simulink model "Control_model_10DOF_fin"  (R2016b)
settings: Solver=FixedStepAuto  StartTime=0.0  StopTime=10  FixedStep=0.0001  RelTol=1e-3
InitFcn:
  | Initialisation_ctr_10DOF_fin
values from neighbouring files (symbols this model uses):
  COM_Parameters = [-lpelvis/2;r2;0]    [Initialisation_ctr_10DOF_fin.m]
  DH_Parameters = [hfoot 0 ... (first row only)    [Initialisation_ctr_10DOF_fin.m]
  dTrunk = trunklbd(3)    [Initialisation_ctr_10DOF_fin.m]
  dxFootSM = dxFoot    [Initialisation_ctr_10DOF_fin.m]
  dxTrunk = 0.1    [Initialisation_ctr_10DOF_fin.m]
  Foot_Parameters = [0;-(lFoot/2-lHeel);0]    [Initialisation_ctr_10DOF_fin.m]
  HAA2HEE = [0; 0; 0.001]    [Initialisation_ctr_10DOF_fin.m]
  HEE2HFE = 0.5*[0.2; 0; 0]    [Initialisation_ctr_10DOF_fin.m]
  height_vrp = CoM_position(1)    [Initialisation_ctr_10DOF_fin.m]
  hTrunk = trunklbd(1)    [Initialisation_ctr_10DOF_fin.m]
  initial_CoM_position = R*CoM_position    [Initialisation_ctr_10DOF_fin.m]
  initial_CoM_velocity = [0;0;0]    [Initialisation_ctr_10DOF_fin.m]
  initial_left_foot = [0;0;-stance_width/2]    [Initialisation_ctr_10DOF_fin.m]
  initial_right_foot = [0;0;stance_width/2]    [Initialisation_ctr_10DOF_fin.m]
  initial_RorL = 0    [Initialisation_ctr_10DOF_fin.m]
  jointsinitial = [9;-15;6;0;0;6;-15;9]/180*pi    [Initialisation_ctr_10DOF_fin.m]
  K_DCM = 4.3*[1 0 0 ... (first row only)    [Initialisation_ctr_10DOF_fin.m]
  kD_left = mbody*[0.95 0 0 0 ... (first row only)    [Initialisation_ctr_10DOF_fin.m]
  kD_right = mbody*[0.12 0 0 0 ... (first row only)    [Initialisation_ctr_10DOF_fin.m]
  kI_left = mbody*[35 0 0 0 ... (first row only)    [Initialisation_ctr_10DOF_fin.m]
  kI_right = mbody*[38.2 0 0 0 ... (first row only)    [Initialisation_ctr_10DOF_fin.m]
  kP_left = mbody*[75 0 0 0 ... (first row only)    [Initialisation_ctr_10DOF_fin.m]
  kP_right = mbody*[5.6 0 0 0 ... (first row only)    [Initialisation_ctr_10DOF_fin.m]
  Lenght = [lShank;lThigh]    [Initialisation_ctr_10DOF_fin.m]
  lFootSM = lFoot    [Initialisation_ctr_10DOF_fin.m]
  lpelvis = wPelvis    [Initialisation_ctr_10DOF_fin.m]
  mass = mbody    (= 60)    [Initialisation_ctr_10DOF_fin.m]
  Masses = [mThigh; mShank; mTrunk]    [Initialisation_ctr_10DOF_fin.m]
  nb_step = 4    [Initialisation_ctr_10DOF_fin.m]
  nb_step_pattern = 20    [Initialisation_ctr_10DOF_fin.m]
  Pelvis_Parameters = [-lpelvis/2;hTrunk/2;0]    [Initialisation_ctr_10DOF_fin.m]
  stance_width = lpelvis    [Initialisation_ctr_10DOF_fin.m]
  stride_lenght = 0.50    (= 0.5)    [Initialisation_ctr_10DOF_fin.m]
  T_DS = time_DS    (= 0.4)    [Initialisation_ctr_10DOF_fin.m]
  T_IT = time_DS    (= 0.4)    [Initialisation_ctr_10DOF_fin.m]
  T_SS = time_swing    (= 1.6)    [Initialisation_ctr_10DOF_fin.m]
  time_DS = (time_stance-time_swing)/2    (= 0.4)    [Initialisation_ctr_10DOF_fin.m]
  time_stance = 60/100*time_stride    (= 2.4)    [Initialisation_ctr_10DOF_fin.m]
  time_step = time_stride/2    (= 2)    [Initialisation_ctr_10DOF_fin.m]
  time_swing = 40/100*time_stride    (= 1.6)    [Initialisation_ctr_10DOF_fin.m]
  validity_angle = [-20*pi/180 20*pi/180 ... (first row only)    [Initialisation_ctr_10DOF_fin.m]
  wTrunk = trunklbd(2)    [Initialisation_ctr_10DOF_fin.m]
  x4CoM = CoM_position(1)-XR4(1)    [Initialisation_ctr_10DOF_fin.m]
undefined symbols (not defined in the file or in its folder): dsegment, hFoot, l, lFoot, omega0_x, omega0_z, rho, wPelvis, X, Xp_x, Xp_z, Y, Z
undefined symbols (not defined in the file): k_grf, lShankSM, lThighSM, mShank, mThigh
libraries: nesl_utility x247, sm_lib x215, dspindex x12, FootPlacementLibrary x8, dspsigops x4, dspswit3 x1
(part 1 of 18)
settings Model: Creator=Damien  LastModifiedBy=Damien

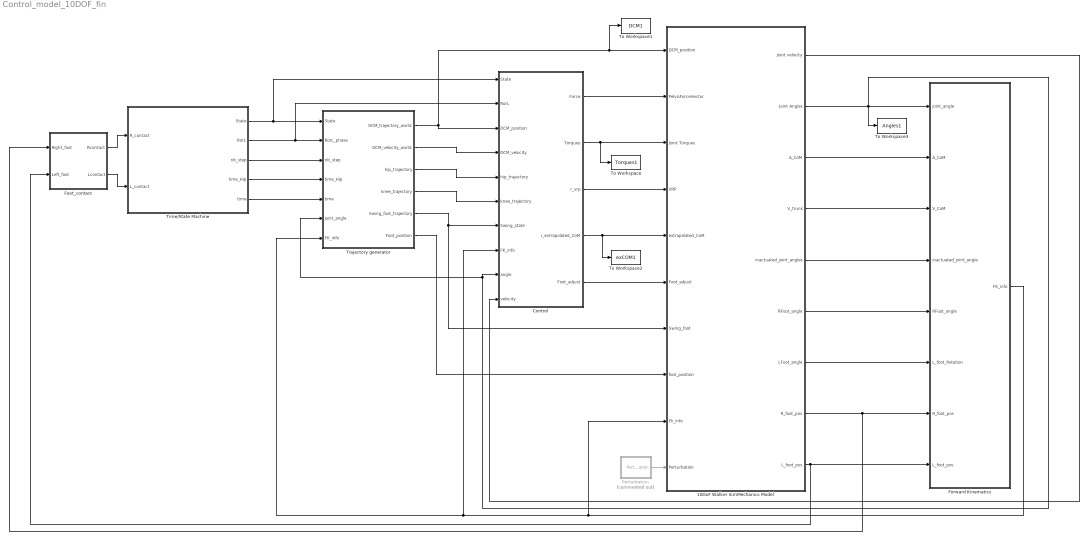
== system Control_model_10DOF_fin ==
  10DoF Walker SimMechanics Model : Subsystem
  Control : Subsystem
  Foot_contact : Subsystem
  Forward Kinematics : Subsystem
  Perturbation : Subsystem  Commented=on
  Time/State Machine : Subsystem
  To Workspace : ToWorkspace  VariableName=Torques1  SaveFormat=Timeseries  SampleTime=-1
  To Workspace1 : ToWorkspace  VariableName=DCM1  SaveFormat=Timeseries  SampleTime=-1
  To Workspace2 : ToWorkspace  VariableName=exCOM1  SaveFormat=Timeseries  SampleTime=-1
  To Workspace3 : ToWorkspace  VariableName=Angles1  SaveFormat=Timeseries  SampleTime=-1
  Trajectory generator : Subsystem
  wires:
  10DoF Walker SimMechanics Model/1(Joint velocity) -> Control/10(velocity)
  10DoF Walker SimMechanics Model/2(Joint Angles) -> Trajectory generator/6(joint_angle), Control/9(angle), To Workspace3/1, Forward Kinematics/1(joint_angle)
  Forward Kinematics/1(FK_info) -> Trajectory generator/7(FK_info), Control/8(FK_info), 10DoF Walker SimMechanics Model/9(Fk_info)
  10DoF Walker SimMechanics Model/4(V_trunk) -> Forward Kinematics/3(V_CoM)
  10DoF Walker SimMechanics Model/6(RFoot_angle) -> Forward Kinematics/5(RFoot_angle)
  10DoF Walker SimMechanics Model/3(A_CoM) -> Forward Kinematics/2(A_CoM)
  10DoF Walker SimMechanics Model/8(R_foot_pos) -> Foot_contact/1(Right_foot), Forward Kinematics/7(R_foot_pos)
  Trajectory generator/5(Swing_foot_trajectory) -> 10DoF Walker SimMechanics Model/7(Swing_foot), Control/7(Swing_state)
  Trajectory generator/1(DCM_trajectory_world) -> To Workspace1/1, 10DoF Walker SimMechanics Model/1(DCM_position), Control/3(DCM_position)
  Trajectory generator/6(Foot_position) -> 10DoF Walker SimMechanics Model/8(foot_position)
  Trajectory generator/2(DCM_velocity_world) -> Control/4(DCM_velocity)
  10DoF Walker SimMechanics Model/7(LFoot_angle) -> Forward Kinematics/6(L_foot_Rotation)
  10DoF Walker SimMechanics Model/9(L_foot_pos) -> Foot_contact/2(Left_foot), Forward Kinematics/8(L_foot_pos)
  10DoF Walker SimMechanics Model/5(inactuated_joint_angles) -> Forward Kinematics/4(inactuated_joint_angle)
  Control/2(Torques) -> 10DoF Walker SimMechanics Model/3(Joint Torques), To Workspace/1
  Control/1(Force) -> 10DoF Walker SimMechanics Model/2(PelvisForceVector)
  Control/3(r_vrp) -> 10DoF Walker SimMechanics Model/4(VRP)
  Control/4(r_extrapolated_CoM) -> 10DoF Walker SimMechanics Model/5(extrapolated_CoM), To Workspace2/1
  Trajectory generator/3(hip_trajectory) -> Control/5(hip_trajectory)
  Time/State Machine/2(RorL) -> Control/2(RorL), Trajectory generator/2(RorL_phase)
  Time/State Machine/3(nb_step) -> Trajectory generator/3(nb_step)
  Time/State Machine/1(State) -> Control/1(State), Trajectory generator/1(State)
  Time/State Machine/4(time_Hip) -> Trajectory generator/4(time_Hip)
  Foot_contact/1(Rcontact) -> Time/State Machine/1(R_contact)
  Foot_contact/2(Lcontact) -> Time/State Machine/2(L_contact)
  Control/5(Foot_adjust) -> 10DoF Walker SimMechanics Model/6(Foot_adjust)
  Time/State Machine/5(time) -> Trajectory generator/5(time)
  Trajectory generator/4(knee_trajectory) -> Control/6(knee_trajectory)
  Perturbation/1(Perturbation) -> 10DoF Walker SimMechanics Model/10(Perturbation)

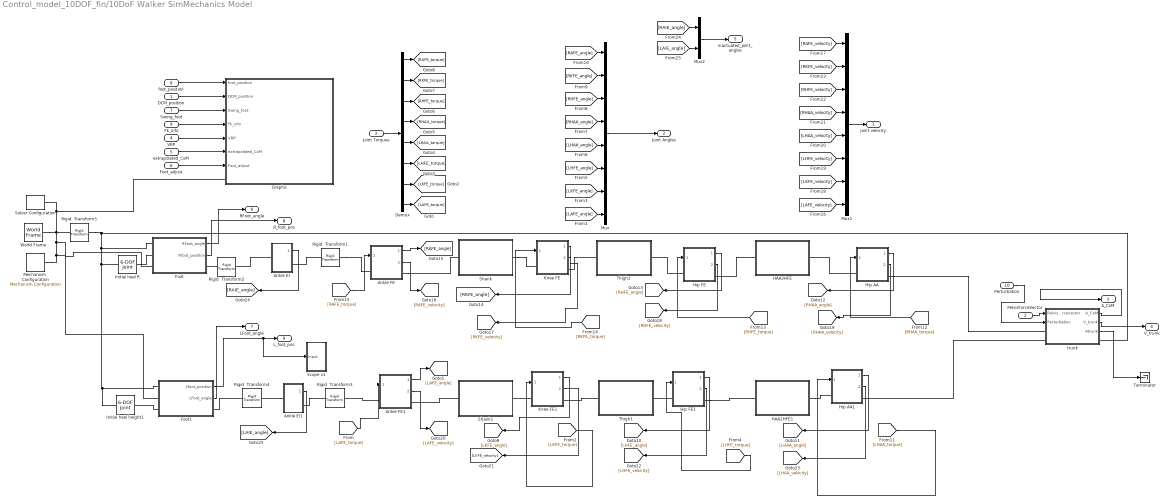
== system Control_model_10DOF_fin/10DoF Walker SimMechanics Model ==
  DCM_position : Inport
  PelvisForceVector : Inport  Port=2
  Joint Torques : Inport  Port=3  PortDimensions=8
  VRP : Inport  Port=4
  extrapolated_CoM : Inport  Port=5
  Foot_adjust : Inport  Port=6
  Swing_foot : Inport  Port=7
  foot_position : Inport  Port=8
  Fk_info : Inport  Port=9
  Perturbation : Inport  Port=10
  Ankle EI : Subsystem
  Ankle EI1 : Subsystem
  Ankle FE : Subsystem
  Ankle FE1 : Subsystem
  Demux : Demux  Outputs=8
  Foot : Subsystem  mask{l=lFootSM, k=k_grf}
      mask prompts: l "Foot length"; k "Ground contact parameters"
  Foot1 : Subsystem  mask{l=lFootSM, k=k_grf}
      mask prompts: l "Foot length"; k "Ground contact parameters"
  Graphic : Subsystem
  HAA2HFE : Subsystem
  HAA2HFE1 : Subsystem
  Hip AA : Subsystem
  Hip AA1 : Subsystem
  Hip FE : Subsystem
  Hip FE1 : Subsystem
  Initial heel R : sm_lib/Joints/6-DOF Joint  SenseConstraintForce=off  SenseConstraintForceX=off  SenseConstraintForceY=off  SenseConstraintForceZ=off  SenseConstraintTorque=off  SenseConstraintTorqueX=off  SenseConstraintTorqueY=off  SenseConstraintTorqueZ=off  SenseTotalForce=off  SenseTotalForceX=off  SenseTotalForceY=off  SenseTotalForceZ=off  SenseTotalTorque=off  SenseTotalTorqueX=off  SenseTotalTorqueY=off  SenseTotalTorqueZ=off  CompositeWrenchDir=FollowerOnBase  CompositeWrenchFrame=BaseFrame  PxEquilibriumPosition=0  PxEquilibriumPositionUnits=m  PxSpringStiffness=0  PxSpringStiffnessUnits=N/m  PxDampingCoefficient=0  PxDampingCoefficientUnits=N/(m/s)  PxTorqueActuationMode=NoTorque  PxMotionActuationMode=ComputedMotion  PxSensePosition=off  PxSenseVelocity=off  PxSenseAcceleration=off  PxSenseTorqueForce=off  PxPositionTargetSpecify=off  PxPositionTargetPriority=High  PxPositionTargetValue=0  PxPositionTargetValueUnits=m  PxVelocityTargetSpecify=off  PxVelocityTargetPriority=High  PxVelocityTargetValue=0  PxVelocityTargetValueUnits=m/s  PyEquilibriumPosition=0  PyEquilibriumPositionUnits=m  PySpringStiffness=0  PySpringStiffnessUnits=N/m  PyDampingCoefficient=0  PyDampingCoefficientUnits=N/(m/s)  PyTorqueActuationMode=NoTorque  PyMotionActuationMode=ComputedMotion  PySensePosition=off  PySenseVelocity=off  PySenseAcceleration=off  PySenseTorqueForce=off  PyPositionTargetSpecify=off  PyPositionTargetPriority=High  PyPositionTargetValue=0  PyPositionTargetValueUnits=m  PyVelocityTargetSpecify=off  PyVelocityTargetPriority=High  PyVelocityTargetValue=0  PyVelocityTargetValueUnits=m/s  PzEquilibriumPosition=0  PzEquilibriumPositionUnits=m  PzSpringStiffness=0  PzSpringStiffnessUnits=N/m  PzDampingCoefficient=0  PzDampingCoefficientUnits=N/(m/s)  PzTorqueActuationMode=NoTorque  PzMotionActuationMode=ComputedMotion  PzSensePosition=off  PzSenseVelocity=off  PzSenseAcceleration=off  PzSenseTorqueForce=off  PzPositionTargetSpecify=off  PzPositionTargetPriority=High  PzPositionTargetValue=0  PzPositionTargetValueUnits=m  PzVelocityTargetSpecify=off  PzVelocityTargetPriority=High  PzVelocityTargetValue=0  PzVelocityTargetValueUnits=m/s  SphDefPosRotationMethod=None  SphDefPosRotationAngleUnits=deg  SphDefPosRotationStandardAxis=+Z  SphDefPosRotationAngle=0  SphDefPosRotationArbitraryAxis=[0 0 1]  SphDefPosFollAlignAxisA=+X  SphDefPosBaseAlignAxisA=+Y  SphDefPosFollAlignAxisB=+Y  SphDefPosBaseAlignAxisB=+Z  SphDefPosRotationSequenceAxes=FollowerAxes  SphDefPosRotationSequence=XYX  SphDefPosRotationSequenceAngles=[0 0 0]  SphDefPosRotationSequenceAnglesUnits=deg  SphDefPosRotationMatrix=[1 0 0; 0 1 0; 0 0 1]  SphEqPosRotationMethod=None  SphEqPosRotationAngleUnits=deg  SphEqPosRotationStandardAxis=+Z  SphEqPosRotationAngle=0  SphEqPosRotationArbitraryAxis=[0 0 1]  SphEqPosFollAlignAxisA=+X  SphEqPosBaseAlignAxisA=+Y  SphEqPosFollAlignAxisB=+Y  SphEqPosBaseAlignAxisB=+Z  SphEqPosRotationSequenceAxes=FollowerAxes  SphEqPosRotationSequence=XYX  SphEqPosRotationSequenceAngles=[0 0 0]  SphEqPosRotationSequenceAnglesUnits=deg  SphEqPosRotationMatrix=[1 0 0; 0 1 0; 0 0 1]  SphSpringStiffness=0  SphSpringStiffnessUnits=N*m/deg  SphDampingCoefficient=0  SphDampingCoefficientUnits=N*m/(deg/s)  SphActuateTorqueX=off  SphActuateTorqueY=off  SphActuateTorqueZ=off  SphActuateTorque=off  SphTorqueActuationMode=NoTorque  SphMotionActuationMode=ComputedMotion  SphActuationFrame=BaseFrame  SphSensePosition=off  SphSenseVelocityX=off  SphSenseVelocityY=off  SphSenseVelocityZ=off  SphSenseVelocity=off  SphSenseAccelerationX=off  SphSenseAccelerationY=off  SphSenseAccelerationZ=off  SphSenseAcceleration=off  SphSenseTorqueX=off  SphSenseTorqueY=off  SphSenseTorqueZ=off  SphSenseTorqueForce=off  SphSensingFrame=BaseFrame  SphPositionTargetRotationMethod=None  SphPositionTargetRotationAngleUnits=deg  SphPositionTargetRotationStandardAxis=+Z  SphPositionTargetRotationAngle=0  SphPositionTargetRotationArbitraryAxis=[0 0 1]  SphPositionTargetFollAlignAxisA=+X  SphPositionTargetBaseAlignAxisA=+Y  SphPositionTargetFollAlignAxisB=+Y  SphPositionTargetBaseAlignAxisB=+Z  SphPositionTargetRotationSequenceAxes=FollowerAxes  SphPositionTargetRotationSequence=XYX  SphPositionTargetRotationSequenceAngles=[0 0 0]  SphPositionTargetRotationSequenceAnglesUnits=deg  SphPositionTargetRotationMatrix=[1 0 0; 0 1 0; 0 0 1]  SphPositionTargetSpecify=off  SphPositionTargetPriority=High  SphVelocityTargetValue=[0 0 0]  SphVelocityTargetValueUnits=deg/s  SphVelocityTargetSpecify=off  SphVelocityTargetPriority=High  SphVelocityTargetInFollowerFrame=on
  Initial heel height1 : sm_lib/Joints/6-DOF Joint  SenseConstraintForce=off  SenseConstraintForceX=off  SenseConstraintForceY=off  SenseConstraintForceZ=off  SenseConstraintTorque=off  SenseConstraintTorqueX=off  SenseConstraintTorqueY=off  SenseConstraintTorqueZ=off  SenseTotalForce=off  SenseTotalForceX=off  SenseTotalForceY=off  SenseTotalForceZ=off  SenseTotalTorque=off  SenseTotalTorqueX=off  SenseTotalTorqueY=off  SenseTotalTorqueZ=off  CompositeWrenchDir=FollowerOnBase  CompositeWrenchFrame=BaseFrame  PxEquilibriumPosition=0  PxEquilibriumPositionUnits=m  PxSpringStiffness=0  PxSpringStiffnessUnits=N/m  PxDampingCoefficient=0  PxDampingCoefficientUnits=N/(m/s)  PxTorqueActuationMode=NoTorque  PxMotionActuationMode=ComputedMotion  PxSensePosition=off  PxSenseVelocity=off  PxSenseAcceleration=off  PxSenseTorqueForce=off  PxPositionTargetSpecify=off  PxPositionTargetPriority=High  PxPositionTargetValue=0  PxPositionTargetValueUnits=m  PxVelocityTargetSpecify=off  PxVelocityTargetPriority=High  PxVelocityTargetValue=0  PxVelocityTargetValueUnits=m/s  PyEquilibriumPosition=0  PyEquilibriumPositionUnits=m  PySpringStiffness=0  PySpringStiffnessUnits=N/m  PyDampingCoefficient=0  PyDampingCoefficientUnits=N/(m/s)  PyTorqueActuationMode=NoTorque  PyMotionActuationMode=ComputedMotion  PySensePosition=off  PySenseVelocity=off  PySenseAcceleration=off  PySenseTorqueForce=off  PyPositionTargetSpecify=on  PyPositionTargetPriority=High  PyPositionTargetValue=0  PyPositionTargetValueUnits=m  PyVelocityTargetSpecify=off  PyVelocityTargetPriority=High  PyVelocityTargetValue=0  PyVelocityTargetValueUnits=m/s  PzEquilibriumPosition=0  PzEquilibriumPositionUnits=m  PzSpringStiffness=0  PzSpringStiffnessUnits=N/m  PzDampingCoefficient=0  PzDampingCoefficientUnits=N/(m/s)  PzTorqueActuationMode=NoTorque  PzMotionActuationMode=ComputedMotion  PzSensePosition=off  PzSenseVelocity=off  PzSenseAcceleration=off  PzSenseTorqueForce=off  PzPositionTargetSpecify=off  PzPositionTargetPriority=High  PzPositionTargetValue=0  PzPositionTargetValueUnits=m  PzVelocityTargetSpecify=off  PzVelocityTargetPriority=High  PzVelocityTargetValue=0  PzVelocityTargetValueUnits=m/s  SphDefPosRotationMethod=None  SphDefPosRotationAngleUnits=deg  SphDefPosRotationStandardAxis=+Z  SphDefPosRotationAngle=0  SphDefPosRotationArbitraryAxis=[0 0 1]  SphDefPosFollAlignAxisA=+X  SphDefPosBaseAlignAxisA=+Y  SphDefPosFollAlignAxisB=+Y  SphDefPosBaseAlignAxisB=+Z  SphDefPosRotationSequenceAxes=FollowerAxes  SphDefPosRotationSequence=XYX  SphDefPosRotationSequenceAngles=[0 0 0]  SphDefPosRotationSequenceAnglesUnits=deg  SphDefPosRotationMatrix=[1 0 0; 0 1 0; 0 0 1]  SphEqPosRotationMethod=None  SphEqPosRotationAngleUnits=deg  SphEqPosRotationStandardAxis=+Z  SphEqPosRotationAngle=0  SphEqPosRotationArbitraryAxis=[0 0 1]  SphEqPosFollAlignAxisA=+X  SphEqPosBaseAlignAxisA=+Y  SphEqPosFollAlignAxisB=+Y  SphEqPosBaseAlignAxisB=+Z  SphEqPosRotationSequenceAxes=FollowerAxes  SphEqPosRotationSequence=XYX  SphEqPosRotationSequenceAngles=[0 0 0]  SphEqPosRotationSequenceAnglesUnits=deg  SphEqPosRotationMatrix=[1 0 0; 0 1 0; 0 0 1]  SphSpringStiffness=0  SphSpringStiffnessUnits=N*m/deg  SphDampingCoefficient=0  SphDampingCoefficientUnits=N*m/(deg/s)  SphActuateTorqueX=off  SphActuateTorqueY=off  SphActuateTorqueZ=off  SphActuateTorque=off  SphTorqueActuationMode=NoTorque  SphMotionActuationMode=ComputedMotion  SphActuationFrame=BaseFrame  SphSensePosition=off  SphSenseVelocityX=off  SphSenseVelocityY=off  SphSenseVelocityZ=off  SphSenseVelocity=off  SphSenseAccelerationX=off  SphSenseAccelerationY=off  SphSenseAccelerationZ=off  SphSenseAcceleration=off  SphSenseTorqueX=off  SphSenseTorqueY=off  SphSenseTorqueZ=off  SphSenseTorqueForce=off  SphSensingFrame=BaseFrame  SphPositionTargetRotationMethod=None  SphPositionTargetRotationAngleUnits=deg  SphPositionTargetRotationStandardAxis=+Z  SphPositionTargetRotationAngle=0  SphPositionTargetRotationArbitraryAxis=[0 0 1]  SphPositionTargetFollAlignAxisA=+X  SphPositionTargetBaseAlignAxisA=+Y  SphPositionTargetFollAlignAxisB=+Y  SphPositionTargetBaseAlignAxisB=+Z  SphPositionTargetRotationSequenceAxes=FollowerAxes  SphPositionTargetRotationSequence=XYX  SphPositionTargetRotationSequenceAngles=[0 0 0]  SphPositionTargetRotationSequenceAnglesUnits=deg  SphPositionTargetRotationMatrix=[1 0 0; 0 1 0; 0 0 1]  SphPositionTargetSpecify=off  SphPositionTargetPriority=High  SphVelocityTargetValue=[0 0 0]  SphVelocityTargetValueUnits=deg/s  SphVelocityTargetSpecify=off  SphVelocityTargetPriority=High  SphVelocityTargetInFollowerFrame=on
  Knee FE : Subsystem
  Knee FE1 : Subsystem
  Mechanism  Configuration : sm_lib/Utilities/Mechanism Configuration  UniformGravity=Constant  GravityVector=[0 -9.81 0]  GravityUnits=m/s^2  LinearizationDelta=0.001
  Mux : Mux  Inputs=8
  Mux1 : Mux  Inputs=8
  Mux2 : Mux  Inputs=2
  Rigid  Transform1 : sm_lib/Frames and Transforms/Rigid Transform  TranslationMethod=None  TranslationStandardOffset=0  TranslationLengthUnit=m  TranslationStandardAxis=+Z  TranslationCartesianOffset=[-l/2 0 0]  TranslationROffset=0  TranslationROffsetUnits=m  TranslationZOffset=0  TranslationZOffsetUnits=m  TranslationThetaOffset=0  TranslationThetaOffsetUnits=deg  RotationMethod=StandardAxis  RotationAngleUnits=deg  RotationStandardAxis=+Y  RotationAngle=90  RotationArbitraryAxis=[0 0 1]  FollAlignAxisA=+X  BaseAlignAxisA=+Y  FollAlignAxisB=+Y  BaseAlignAxisB=+Z  RotationSequenceAxes=FollowerAxes  RotationSequence=XYX  RotationSequenceAngles=[0 0 0]  RotationSequenceAnglesUnits=deg  RotationMatrix=[1 0 0; 0 1 0; 0 0 1]
  Rigid  Transform2 : sm_lib/Frames and Transforms/Rigid Transform  TranslationMethod=None  TranslationStandardOffset=0  TranslationLengthUnit=m  TranslationStandardAxis=+Z  TranslationCartesianOffset=[-l/2 0 0]  TranslationROffset=0  TranslationROffsetUnits=m  TranslationZOffset=0  TranslationZOffsetUnits=m  TranslationThetaOffset=0  TranslationThetaOffsetUnits=deg  RotationMethod=StandardAxis  RotationAngleUnits=deg  RotationStandardAxis=+Y  RotationAngle=-90  RotationArbitraryAxis=[0 0 1]  FollAlignAxisA=+X  BaseAlignAxisA=+Y  FollAlignAxisB=+Y  BaseAlignAxisB=+Z  RotationSequenceAxes=FollowerAxes  RotationSequence=XYX  RotationSequenceAngles=[0 0 0]  RotationSequenceAnglesUnits=deg  RotationMatrix=[1 0 0; 0 1 0; 0 0 1]
  Rigid  Transform3 : sm_lib/Frames and Transforms/Rigid Transform  TranslationMethod=None  TranslationStandardOffset=0  TranslationLengthUnit=m  TranslationStandardAxis=+Z  TranslationCartesianOffset=[-l/2 0 0]  TranslationROffset=0  TranslationROffsetUnits=m  TranslationZOffset=0  TranslationZOffsetUnits=m  TranslationThetaOffset=0  TranslationThetaOffsetUnits=deg  RotationMethod=StandardAxis  RotationAngleUnits=deg  RotationStandardAxis=+Y  RotationAngle=-90  RotationArbitraryAxis=[0 0 1]  FollAlignAxisA=+X  BaseAlignAxisA=+Y  FollAlignAxisB=+Y  BaseAlignAxisB=+Z  RotationSequenceAxes=FollowerAxes  RotationSequence=XYX  RotationSequenceAngles=[0 0 0]  RotationSequenceAnglesUnits=deg  RotationMatrix=[1 0 0; 0 1 0; 0 0 1]
  Rigid  Transform4 : sm_lib/Frames and Transforms/Rigid Transform  TranslationMethod=None  TranslationStandardOffset=0  TranslationLengthUnit=m  TranslationStandardAxis=+Z  TranslationCartesianOffset=[-l/2 0 0]  TranslationROffset=0  TranslationROffsetUnits=m  TranslationZOffset=0  TranslationZOffsetUnits=m  TranslationThetaOffset=0  TranslationThetaOffsetUnits=deg  RotationMethod=StandardAxis  RotationAngleUnits=deg  RotationStandardAxis=+Y  RotationAngle=90  RotationArbitraryAxis=[0 0 1]  FollAlignAxisA=+X  BaseAlignAxisA=+Y  FollAlignAxisB=+Y  BaseAlignAxisB=+Z  RotationSequenceAxes=FollowerAxes  RotationSequence=XYX  RotationSequenceAngles=[0 0 0]  RotationSequenceAnglesUnits=deg  RotationMatrix=[1 0 0; 0 1 0; 0 0 1]
  Rigid  Transform5 : sm_lib/Frames and Transforms/Rigid Transform  TranslationMethod=Cartesian  TranslationStandardOffset=0  TranslationLengthUnit=m  TranslationStandardAxis=+Z  TranslationCartesianOffset=[-lFootSM/2 0 -lpelvis/2]  TranslationROffset=0  TranslationROffsetUnits=m  TranslationZOffset=0  TranslationZOffsetUnits=m  TranslationThetaOffset=0  TranslationThetaOffsetUnits=deg  RotationMethod=None  RotationAngleUnits=deg  RotationStandardAxis=+Y  RotationAngle=90  RotationArbitraryAxis=[0 0 1]  FollAlignAxisA=+X  BaseAlignAxisA=+Y  FollAlignAxisB=+Y  BaseAlignAxisB=+Z  RotationSequenceAxes=FollowerAxes  RotationSequence=XYX  RotationSequenceAngles=[0 0 0]  RotationSequenceAnglesUnits=deg  RotationMatrix=[1 0 0; 0 1 0; 0 0 1]
  Scope x1 : Subsystem
  Shank : Subsystem  mask{l=lShankSM, m=mShank}
      mask prompts: l "Shank length"; m "Shank mass"
  Shank1 : Subsystem  mask{l=lShankSM, m=mShank}
      mask prompts: l "Shank length"; m "Shank mass"
  Solver Configuration : nesl_utility/Solver Configuration  PhysicalDomain=network_engine_domain  SubClassName=solver  LeftPortType=input  RightPortType=generic  Accelerate=off  Tones=[]  Harmonics=[]  SimulateNoise=off  Profile=off  UseLocalSampling=off  EnableSwitchedLinearOptims=on  FrequencyDomain=off  UseCCode=off  RelTol=0.001  AbsTol=1e-06  MinStep=1e-09  ToWorkspace=off  RevertToSquareIcSolve=off  NumHomotopyIterations=100  PhasorMode=off  PhasorModeNumHarmonics=1  OverrideAbsTol=off  DoDC=off  ResidualTolerance=1e-09  UseLocalSolver=off  LocalSolverChoice=NE_BACKWARD_EULER_ADVANCER  LocalSolverSampleTime=0.001  DoFixedCost=off  MaxNonlinIter=3  MaxModeIter=2  LinearAlgebra=Sparse  DelaysMemoryBudget=1024  AutomaticFiltering=on  FilteringTimeConstant=0.001
  Terminator : Terminator
  Thigh1 : Subsystem  mask{l=lThighSM, m=mThigh}
      mask prompts: l "Thigh length [m]"; m "Thigh mass [kg]"
  Thigh2 : Subsystem  mask{l=lThighSM, m=mThigh}
      mask prompts: l "Thigh length [m]"; m "Thigh mass [kg]"
  World Frame : sm_lib/Frames and Transforms/World Frame
  trunk : Subsystem
  Joint velocity : Outport  Unit=rad/s  PortDimensions=8
  Joint Angles : Outport  Port=2  Unit=rad  PortDimensions=8
  A_CoM : Outport  Port=3
  V_trunk : Outport  Port=4
  inactuated_joint_angles : Outport  Port=5
  RFoot_angle : Outport  Port=6
  LFoot_angle : Outport  Port=7
  R_foot_pos : Outport  Port=8
  L_foot_pos : Outport  Port=9
  wires:
  trunk/1(A_CoM) -> A_CoM/1
  PelvisForceVector/1 -> trunk/1(PelvisForceVector)
  Joint Torques/1 -> Demux/1
  Mux/1 -> Joint Angles/1
  [LAFE_torque] -> Ankle FE1/1(torque)
  Ankle FE1/1(position) -> [LAFE_angle]
  [LKFE_torque] -> Knee FE1/1(torque)
  Knee FE1/1(position) -> [LKFE_angle]
  [LHFE_torque] -> Hip FE1/1(torque)
  Hip FE1/1(position) -> [LHFE_angle]
  [LHAA_torque] -> Hip AA1/1(torque)
  Hip AA1/1(position) -> [LHAA_angle]
  Hip AA/1(position) -> [RHAA_angle]
  Knee FE/1(position) -> [RKFE_angle]
  Mux1/1 -> Joint velocity/1
  Knee FE/2(velocity) -> [RKFE_velocity]
  Hip FE/1(position) -> [RHFE_angle]
  Hip AA/2(velocity) -> [RHAA_velocity]
  Ankle FE1/2(velocity) -> [LAFE_velocity]
  Knee FE1/2(velocity) -> [LKFE_velocity]
  Hip AA1/2(velocity) -> [LHAA_velocity]
  Demux/8 -> [LAFE_torque]
  Demux/7 -> [LKFE_torque]
  Demux/6 -> [LHFE_torque]
  Demux/5 -> [LHAA_torque]
  Demux/4 -> [RHAA_torque]
  Demux/3 -> [RHFE_torque]
  Demux/2 -> [RKFE_torque]
  Demux/1 -> [RAFE_torque]
  [LAFE_angle] -> Mux/8
  [LKFE_angle] -> Mux/7
  [LHFE_angle] -> Mux/6
  [LHAA_angle] -> Mux/5
  [RHAA_angle] -> Mux/4
  [RHFE_angle] -> Mux/3
  [RKFE_angle] -> Mux/2
  [RAFE_angle] -> Mux/1
  [LAFE_velocity] -> Mux1/8
  [RAFE_velocity] -> Mux1/1
  [LKFE_velocity] -> Mux1/7
  [LHFE_velocity] -> Mux1/6
  [LHAA_velocity] -> Mux1/5
  [RHAA_velocity] -> Mux1/4
  [RHFE_velocity] -> Mux1/3
  [RKFE_velocity] -> Mux1/2
  Fk_info/1 -> Graphic/4(Fk_info)
  Mux2/1 -> inactuated_joint_angles/1
  [RAIE_angle] -> Mux2/1
  [LAIE_angle] -> Mux2/2
  Ankle EI1/1(position) -> [LAIE_angle]
  Foot/1(RFoot_angle) -> RFoot_angle/1
  trunk/2(V_trunk) -> V_trunk/1
  Foot/2(Rfoot_position) -> R_foot_pos/1
  Swing_foot/1 -> Graphic/3(Swing_foot)
  DCM_position/1 -> Graphic/2(DCM_position)
  foot_position/1 -> Graphic/1(foot_position)
  VRP/1 -> Graphic/5(VRP)
  extrapolated_CoM/1 -> Graphic/6(extrapolated_CoM)
  Foot1/1(Lfoot_position) -> Scope x1/1(Input), L_foot_pos/1
  Foot1/2(LFoot_angle) -> LFoot_angle/1
  Foot_adjust/1 -> Graphic/7(Foot_adjust)
  Ankle EI/1(position) -> [RAIE_angle]
  [RAFE_torque] -> Ankle FE/1(torque)
  Ankle FE/1(position) -> [RAFE_angle]
  Ankle FE/2(velocity) -> [RAFE_velocity]
  [RKFE_torque] -> Knee FE/1(torque)
  [RHFE_torque] -> Hip FE/1(torque)
  Hip FE/2(velocity) -> [RHFE_velocity]
  Hip FE1/2(velocity) -> [LHFE_velocity]
  [RHAA_torque] -> Hip AA/1(torque)
  Perturbation/1 -> trunk/2(Perturbation)
  trunk/3(Rtrunk) -> Terminator/1
  connections:
  Foot/LConn1 -- Rigid  Transform5/RConn1 -- trunk/RConn1 -- Initial heel R/LConn1 -- Initial heel height1/LConn1 -- Foot1/LConn1
  Shank1/LConn1 -- Ankle FE1/RConn1
  Foot1/LConn3 -- Initial heel height1/RConn1
  Foot/LConn2 -- Initial heel R/RConn1
  Knee FE/RConn1 -- Thigh2/LConn1
  Rigid  Transform2/LConn1 -- Foot/RConn1
  Ankle FE1/LConn1 -- Rigid  Transform3/RConn1
  Rigid  Transform4/LConn1 -- Foot1/RConn1
  Ankle EI1/LConn1 -- Rigid  Transform4/RConn1
  Ankle EI1/RConn1 -- Rigid  Transform3/LConn1
  Mechanism  Configuration/RConn1 -- Foot1/LConn2 -- Foot/LConn3 -- Rigid  Transform5/LConn1 -- World Frame/RConn1 -- Graphic/LConn1 -- Solver Configuration/RConn1
  Ankle EI/RConn1 -- Rigid  Transform1/LConn1
  Ankle EI/LConn1 -- Rigid  Transform2/RConn1
  Rigid  Transform1/RConn1 -- Ankle FE/LConn1
  Ankle FE/RConn1 -- Shank/LConn1
  Shank/RConn1 -- Knee FE/LConn1
  Knee FE1/LConn1 -- Shank1/RConn1
  Knee FE1/RConn1 -- Thigh1/LConn1
  Hip FE/LConn1 -- Thigh2/RConn1
  Hip FE/RConn1 -- HAA2HFE/LConn1
  Hip FE1/LConn1 -- Thigh1/RConn1
  Hip FE1/RConn1 -- HAA2HFE1/LConn1
  Hip AA/RConn1 -- trunk/LConn1
  Hip AA/LConn1 -- HAA2HFE/RConn1
  HAA2HFE1/RConn1 -- Hip AA1/LConn1
  Hip AA1/RConn1 -- trunk/LConn2

== system Control_model_10DOF_fin/Control ==
  State : Inport
  RorL : Inport  Port=2
  DCM_position : Inport  Port=3
  DCM_velocity : Inport  Port=4
  hip_trajectory : Inport  Port=5
  knee_trajectory : Inport  Port=6
  Swing_state : Inport  Port=7
  FK_info : Inport  Port=8
  angle : Inport  Port=9
  velocity : Inport  Port=10
  Double_Support : Subsystem  TreatAsAtomicUnit=on
  Finish_Swing_Phase : Subsystem  TreatAsAtomicUnit=on
  Inititial_Transfert : Subsystem  TreatAsAtomicUnit=on
  Memory3 : Memory  X0=-1
  Merge{1..5} (5 alike) : Merge  Inputs=5
  Relational Operator : RelationalOperator  Operator=~=  OutDataTypeStr=boolean  RndMeth=Simplest
  Sample and Hold1 : dspsigops/Sample and Hold  trig=Falling edge  initCond=0  latchinput=on
  Saturation : Saturate  UpperLimit=250  LowerLimit=-250
  Single_Support : Subsystem  TreatAsAtomicUnit=on
  Stance_position : Subsystem  TreatAsAtomicUnit=on
  Switch Case : SwitchCase  CaseConditions={0,1,2,3,4}  ShowDefaultCase=off
  Force : Outport
  Torques : Outport  Port=2
  r_vrp : Outport  Port=3
  r_extrapolated_CoM : Outport  Port=4  PortDimensions=3
  Foot_adjust : Outport  Port=5
  wires:
  velocity/1 -> Double_Support/6(joint_velocity), Finish_Swing_Phase/6(joint_velocity), Stance_position/2(velocity), Inititial_Transfert/6(joint_velocity), Single_Support/6(joint_velocity)
  angle/1 -> Double_Support/5(joint_angle), Finish_Swing_Phase/5(joint_angle), Single_Support/5(joint_angle), Inititial_Transfert/5(joint_angle), Stance_position/1(angle)
  State/1 -> Memory3/1, Relational Operator/1, Switch Case/1
  Merge4/1 -> Saturation/1
  Switch Case/1 -> Stance_position/Action
  Switch Case/2 -> Inititial_Transfert/Action
  Switch Case/3 -> Single_Support/Action
  Switch Case/4 -> Finish_Swing_Phase/Action
  Switch Case/5 -> Double_Support/Action
  RorL/1 -> Finish_Swing_Phase/1(RorL), Double_Support/1(RorL), Single_Support/1(RorL), Inititial_Transfert/1(RorL)
  DCM_position/1 -> Inititial_Transfert/2(DCM_position), Double_Support/2(DCM_position), Finish_Swing_Phase/2(DCM_position), Single_Support/2(DCM_position)
  DCM_velocity/1 -> Inititial_Transfert/3(DCM_velocity), Single_Support/3(DCM_velocity), Double_Support/3(DCM_velocity), Finish_Swing_Phase/3(DCM_velocity)
  FK_info/1 -> Double_Support/4(FK_info), Finish_Swing_Phase/4(FK_info), Single_Support/4(FK_info), Inititial_Transfert/4(FK_info)
  Swing_state/1 -> Sample and Hold1/1, Single_Support/7(swing_state)
  hip_trajectory/1 -> Inititial_Transfert/7(hip_trajectory), Single_Support/8(hip_trajectory), Double_Support/7(hip_trajectory), Finish_Swing_Phase/8(hip_trajectory)
  Merge1/1 -> Force/1
  Stance_position/2(Torques) -> Merge4/1
  Inititial_Transfert/2(Torques) -> Merge4/2
  Single_Support/2(Torques) -> Merge4/3
  Finish_Swing_Phase/2(Torques) -> Merge4/4
  Double_Support/2(Torques) -> Merge4/5
  Stance_position/1(Force) -> Merge1/1
  Inititial_Transfert/1(Force) -> Merge1/2
  Single_Support/1(Force) -> Merge1/3
  Finish_Swing_Phase/1(Force) -> Merge1/4
  Double_Support/1(Force) -> Merge1/5
  Merge2/1 -> r_vrp/1
  Stance_position/3(r_vrp) -> Merge2/1
  Inititial_Transfert/3(r_vrp) -> Merge2/2
  Single_Support/3(r_vrp) -> Merge2/3
  Finish_Swing_Phase/3(r_vrp) -> Merge2/4
  Double_Support/3(r_vrp) -> Merge2/5
  Merge3/1 -> r_extrapolated_CoM/1
  Stance_position/4(r_extrapolated_CoM) -> Merge3/1
  Inititial_Transfert/4(r_extrapolated_CoM) -> Merge3/2
  Single_Support/4(r_extrapolated_CoM) -> Merge3/3
  Finish_Swing_Phase/4(r_extrapolated_CoM) -> Merge3/4
  Double_Support/4(r_extrapolated_CoM) -> Merge3/5
  Relational Operator/1 -> Sample and Hold1/Trigger
  Memory3/1 -> Relational Operator/2
  Sample and Hold1/1 -> Finish_Swing_Phase/7(swing_state)
  Merge5/1 -> Foot_adjust/1
  Double_Support/5(Foot_adjust) -> Merge5/5
  Finish_Swing_Phase/5(Foot_adjust) -> Merge5/4
  Single_Support/5(Foot_adjust) -> Merge5/3
  Inititial_Transfert/5(Foot_adjust) -> Merge5/2
  Stance_position/5(Foot_adjust) -> Merge5/1
  Saturation/1 -> Torques/1
  knee_trajectory/1 -> Double_Support/8(knee_trajectory), Single_Support/9(knee_trajectory), Finish_Swing_Phase/9(knee_trajectory)

== system Control_model_10DOF_fin/Foot_contact ==
  Right_foot : Inport
  Left_foot : Inport  Port=2
  Constant : Constant  Value=0
  Constant1 : Constant  Value=0
  Relational Operator : RelationalOperator  Operator=<=  OutDataTypeStr=boolean  RndMeth=Simplest
  Relational Operator1 : RelationalOperator  Operator=<=  OutDataTypeStr=boolean  RndMeth=Simplest
  Scope : Scope
  Scope1 : Scope
  Selector : Selector  InputPortWidth=3  IndexOptions=Index vector (dialog)  Indices=[2]  OutputSizes=1
  Selector1 : Selector  InputPortWidth=3  IndexOptions=Index vector (dialog)  Indices=[2]  OutputSizes=1
  Rcontact : Outport
  Lcontact : Outport  Port=2
  wires:
  Right_foot/1 -> Selector/1
  Constant/1 -> Relational Operator/2
  Relational Operator/1 -> Scope/1, Rcontact/1
  Left_foot/1 -> Selector1/1
  Constant1/1 -> Relational Operator1/2
  Relational Operator1/1 -> Scope1/1, Lcontact/1
  Selector/1 -> Relational Operator/1
  Selector1/1 -> Relational Operator1/1

== system Control_model_10DOF_fin/Forward Kinematics ==
  joint_angle : Inport
  A_CoM : Inport  Port=2
  V_CoM : Inport  Port=3
  inactuated_joint_angle : Inport  Port=4
  RFoot_angle : Inport  Port=5
  L_foot_Rotation : Inport  Port=6
  R_foot_pos : Inport  Port=7
  L_foot_pos : Inport  Port=8
  Bus Creator : BusCreator  Inputs=56
  Forward Kinematics : MATLAB Function  TreatAsAtomicUnit=on
  Memory : Memory  X0=[0;0;0]
  FK_info : Outport
  wires:
  joint_angle/1 -> Forward Kinematics/1(joint_angle)
  Bus Creator/1 -> FK_info/1
  V_CoM/1 -> Forward Kinematics/3(V_CoM)
  inactuated_joint_angle/1 -> Forward Kinematics/2(inactuated_joint_angle)
  RFoot_angle/1 -> Forward Kinematics/4(R_foot_Rotation)
  R_foot_pos/1 -> Forward Kinematics/5(R_foot_pos)
  L_foot_Rotation/1 -> Forward Kinematics/6(L_foot_Rotation)
  L_foot_pos/1 -> Forward Kinematics/7(L_foot_pos)
  Forward Kinematics/1(TR0) -> Bus Creator/1
  Forward Kinematics/2(TR1) -> Bus Creator/2
  Forward Kinematics/3(TR2) -> Bus Creator/3
  Forward Kinematics/4(TR3) -> Bus Creator/4
  Forward Kinematics/5(TR4) -> Bus Creator/5
  Forward Kinematics/6(TR5) -> Bus Creator/6
  Forward Kinematics/7(TR6) -> Bus Creator/7
  Forward Kinematics/8(TR7) -> Bus Creator/8
  Forward Kinematics/9(TR8) -> Bus Creator/9
  Forward Kinematics/10(TR9) -> Bus Creator/10
  Forward Kinematics/11(TRL) -> Bus Creator/11
  Forward Kinematics/12(TRthighR) -> Bus Creator/12
  Forward Kinematics/13(TRshankR) -> Bus Creator/13
  Forward Kinematics/14(TRtrunk) -> Bus Creator/14
  Forward Kinematics/15(TRshankL) -> Bus Creator/15
  Forward Kinematics/16(TRthighL) -> Bus Creator/16
  Forward Kinematics/17(TL9) -> Bus Creator/17
  Forward Kinematics/18(TL8) -> Bus Creator/18
  Forward Kinematics/19(TL7) -> Bus Creator/19
  Forward Kinematics/20(TL6) -> Bus Creator/20
  Forward Kinematics/21(TL5) -> Bus Creator/21
  Forward Kinematics/22(TL4) -> Bus Creator/22
  Forward Kinematics/23(TL3) -> Bus Creator/23
  Forward Kinematics/24(TL2) -> Bus Creator/24
  Forward Kinematics/25(TL1) -> Bus Creator/25
  Forward Kinematics/26(TL0) -> Bus Creator/26
  Forward Kinematics/27(TLR) -> Bus Creator/27
  Forward Kinematics/28(TLthighL) -> Bus Creator/28
  Forward Kinematics/29(TLshankL) -> Bus Creator/29
  Forward Kinematics/30(TLtrunk) -> Bus Creator/30
  Forward Kinematics/31(TLshankR) -> Bus Creator/31
  Forward Kinematics/32(TLthighR) -> Bus Creator/32
  Forward Kinematics/33(TWR) -> Bus Creator/33
  Forward Kinematics/34(TWL) -> Bus Creator/34
  Forward Kinematics/35(TW0) -> Bus Creator/35
  Forward Kinematics/36(TW1) -> Bus Creator/36
  Forward Kinematics/37(TW2) -> Bus Creator/37
  Forward Kinematics/38(TW3) -> Bus Creator/38
  Forward Kinematics/39(TW4) -> Bus Creator/39
  Forward Kinematics/40(TW5) -> Bus Creator/40
  Forward Kinematics/41(TW6) -> Bus Creator/41
  Forward Kinematics/42(TW7) -> Bus Creator/42
  Forward Kinematics/43(TW8) -> Bus Creator/43
  Forward Kinematics/44(TW9) -> Bus Creator/44
  Forward Kinematics/45(TWthighR) -> Bus Creator/45
  Forward Kinematics/46(TWthighL) -> Bus Creator/46
  Forward Kinematics/47(TWshankR) -> Bus Creator/47
  Forward Kinematics/48(TWshankL) -> Bus Creator/48
  Forward Kinematics/49(TWtrunk) -> Bus Creator/49
  Forward Kinematics/50(XRcom) -> Bus Creator/50
  Forward Kinematics/51(XLcom) -> Bus Creator/51
  Forward Kinematics/52(XWcom) -> Bus Creator/52
  Forward Kinematics/53(VWcom) -> Bus Creator/53
  A_CoM/1 -> Memory/1
  Forward Kinematics/54(AWcom) -> Bus Creator/54
  Forward Kinematics/55(JRcom) -> Bus Creator/55
  Forward Kinematics/56(JLcom) -> Bus Creator/56
  Memory/1 -> Forward Kinematics/8(A_CoM)

== system Control_model_10DOF_fin/Perturbation ==
  Clock1 : Clock
  Constant : Constant  Value=5.5
  Constant1 : Constant  Value=0.05
  Constant2 : Constant  Commented=on  Value=4.7
  Force : Subsystem  TreatAsAtomicUnit=on
  Force1 : Subsystem  TreatAsAtomicUnit=on
  If Left swing phase : If  IfExpression=u1 ==1
  Logical Operator : Logic  AllPortsSameDT=off  OutDataTypeStr=boolean
  Merge1 : Merge
  Relational Operator1 : RelationalOperator  OutDataTypeStr=boolean  RndMeth=Simplest
  Relational Operator2 : RelationalOperator  Operator=<=  OutDataTypeStr=boolean  RndMeth=Simplest
  Scope{,1..3} (4 alike) : Scope
  Sum1 : Sum  Inputs=|++
  Perturbation : Outport
  wires:
  Merge1/1 -> Scope/1, Perturbation/1
  Clock1/1 -> Relational Operator1/1, Relational Operator2/1
  Constant/1 -> Sum1/1, Relational Operator1/2
  If Left swing phase/2 -> Force1/Action
  If Left swing phase/1 -> Force/Action
  Force/1(perturbation) -> Merge1/1
  Force1/1(perturbation) -> Merge1/2
  Sum1/1 -> Relational Operator2/2
  Constant1/1 -> Sum1/2
  Relational Operator2/1 -> Scope2/1, Logical Operator/2
  Relational Operator1/1 -> Scope1/1, Logical Operator/1
  Logical Operator/1 -> Scope3/1, If Left swing phase/1

== system Control_model_10DOF_fin/Time//State Machine ==
  R_contact : Inport
  L_contact : Inport  Port=2
  Chart : Stateflow chart  TreatAsAtomicUnit=on
  Clock : Clock
  Clock1 : Clock
  Constant : Constant  Value=3
  Hip_timer : Subsystem
  Logical Operator : Logic  AllPortsSameDT=off  OutDataTypeStr=boolean
  Memory : Memory
  Memory1 : Memory
  Relational Operator1 : RelationalOperator  Operator=~=  OutDataTypeStr=boolean  RndMeth=Simplest
  Relational Operator2 : RelationalOperator  Operator=~=  OutDataTypeStr=boolean  RndMeth=Simplest
  Sample and Hold : dspsigops/Sample and Hold  trig=Rising edge  initCond=0  latchinput=on
  Step counter : Subsystem
  Sum1 : Sum  Inputs=|+-
  To Workspace3 : ToWorkspace  VariableName=State  SaveFormat=Timeseries  SampleTime=-1
  State : Outport
  RorL : Outport  Port=2
  nb_step : Outport  Port=3
  time_Hip : Outport  Port=4
  time : Outport  Port=5
  wires:
  Clock1/1 -> Sample and Hold/1
  L_contact/1 -> Chart/3(L_contact)
  Chart/2(RorL) -> Hip_timer/3(RorL), RorL/1
  Memory1/1 -> Chart/1(t)
  Memory/1 -> Relational Operator1/2
  Clock/1 -> Sum1/1
  R_contact/1 -> Chart/2(R_contact)
  Sample and Hold/1 -> Sum1/2
  Sum1/1 -> Hip_timer/2(time), time/1, Memory1/1
  Chart/1(State) -> Hip_timer/1(State), Step counter/1(state), State/1, To Workspace3/1, Relational Operator2/1, Memory/1, Relational Operator1/1
  Hip_timer/1(time_Hip) -> time_Hip/1
  Relational Operator1/1 -> Logical Operator/1
  Relational Operator2/1 -> Logical Operator/2
  Constant/1 -> Relational Operator2/2
  Logical Operator/1 -> Sample and Hold/Trigger
  Step counter/1(nb_step) -> nb_step/1

== system Control_model_10DOF_fin/Trajectory generator ==
  State : Inport  PortDimensions=1
  RorL_phase : Inport  Port=2
  nb_step : Inport  Port=3  PortDimensions=1
  time_Hip : Inport  Port=4  PortDimensions=1
  time : Inport  Port=5
  joint_angle : Inport  Port=6
  FK_info : Inport  Port=7
  Constant : Constant  Value=3
  DCM trajectory : Subsystem
  Enabled and Triggered Subsystem 1 : Subsystem  TreatAsAtomicUnit=on
  Hip trajectory2 : Subsystem
  Logical Operator : Logic  AllPortsSameDT=off  OutDataTypeStr=boolean
  Memory3 : Memory  X0=-1
  Relational Operator : RelationalOperator  Operator=~=  OutDataTypeStr=boolean  RndMeth=Simplest
  Relational Operator1 : RelationalOperator  Operator=~=  OutDataTypeStr=boolean  RndMeth=Simplest
  Subsystem1 : Subsystem
  Terminator : Terminator
  first_foot (init swing foot) : Selector  InputPortWidth=3*(nb_step)  IndexOptions=Index vector (dialog)  Indices=[1 2 3]  OutputSizes=1
  knee trajectory : Subsystem
  second_foot (stance foot position) : Selector  InputPortWidth=3*(nb_step)  IndexOptions=Index vector (dialog)  Indices=[4 5 6]  OutputSizes=1
  third_foot (end swing foot) : Selector  InputPortWidth=3*(nb_step)  IndexOptions=Index vector (dialog)  Indices=[7 8 9]  OutputSizes=1
  DCM_trajectory_world : Outport  OutDataTypeStr=double  Unit=m  PortDimensions=3
  DCM_velocity_world : Outport  Port=2  OutDataTypeStr=double  Unit=m/s  PortDimensions=3
  hip_trajectory : Outport  Port=3
  knee_trajectory : Outport  Port=4
  Swing_foot_trajectory : Outport  Port=5
  Foot_position : Outport  Port=6
  wires:
  Enabled and Triggered Subsystem 1/1(feet_positions) -> Foot_position/1, first_foot (init swing foot)/1, third_foot (end swing foot)/1, second_foot (stance foot position)/1, DCM trajectory/1(feet_positions)
  DCM trajectory/2(DCM_velocity) -> DCM_velocity_world/1
  first_foot (init swing foot)/1 -> Subsystem1/1(foot_position_ini)
  third_foot (end swing foot)/1 -> Subsystem1/2(foot_position_fin)
  RorL_phase/1 -> knee trajectory/4(RorL_phase), Enabled and Triggered Subsystem 1/3(RorL)
  nb_step/1 -> Hip trajectory2/3(nb_step), Enabled and Triggered Subsystem 1/1(nb_step)
  Memory3/1 -> Relational Operator/2
  FK_info/1 -> Enabled and Triggered Subsystem 1/2(FK_info)
  DCM trajectory/1(DCM_position) -> DCM_trajectory_world/1
  Subsystem1/1(swing_foot_trajectory) -> Swing_foot_trajectory/1
  second_foot (stance foot position)/1 -> Terminator/1
  Hip trajectory2/1(hip_trajectory) -> hip_trajectory/1
  State/1 -> Relational Operator1/2, Relational Operator/1, Memory3/1, Enabled and Triggered Subsystem 1/4(State), Hip trajectory2/1(State), Subsystem1/4(State), knee trajectory/2(State), DCM trajectory/3(State)
  time_Hip/1 -> Hip trajectory2/2(time_Hip)
  time/1 -> Subsystem1/3(time), knee trajectory/1(time), DCM trajectory/2(time)
  Relational Operator/1 -> Logical Operator/2
  Logical Operator/1 -> Enabled and Triggered Subsystem 1/Trigger
  Relational Operator1/1 -> Logical Operator/1
  Constant/1 -> Relational Operator1/1
  knee trajectory/1(knee_trajectory) -> knee_trajectory/1
  joint_angle/1 -> knee trajectory/3(joint_angle)

== system Control_model_10DOF_fin/10DoF Walker SimMechanics Model/Ankle EI ==
  Ankle Joint2 : sm_lib/Joints/Revolute Joint  SenseConstraintForce=off  SenseConstraintForceX=off  SenseConstraintForceY=off  SenseConstraintForceZ=off  SenseConstraintTorque=off  SenseConstraintTorqueX=off  SenseConstraintTorqueY=off  SenseConstraintTorqueZ=off  SenseTotalForce=off  SenseTotalForceX=off  SenseTotalForceY=off  SenseTotalForceZ=off  SenseTotalTorque=off  SenseTotalTorqueX=off  SenseTotalTorqueY=off  SenseTotalTorqueZ=off  CompositeWrenchDir=FollowerOnBase  CompositeWrenchFrame=BaseFrame  EquilibriumPosition=0  EquilibriumPositionUnits=deg  SpringStiffness=ankle_stiffness  SpringStiffnessUnits=N*m/rad  DampingCoefficient=joint_damping  DampingCoefficientUnits=N*m/(rad/s)  TorqueActuationMode=InputTorque  MotionActuationMode=ComputedMotion  SensePosition=on  SenseVelocity=off  SenseAcceleration=off  SenseTorqueForce=off  PositionTargetSpecify=on  PositionTargetPriority=High  PositionTargetValue=0  PositionTargetValueUnits=deg  VelocityTargetSpecify=off  VelocityTargetPriority=High  VelocityTargetValue=0  VelocityTargetValueUnits=deg/s
  Conv17 : nesl_utility/PS-Simulink Converter  PhysicalDomain=network_engine_domain  SubClassName=ps_output  LeftPortType=input  RightPortType=output  PseudoPeriodic=off  Frequencies=[]  Unit=rad  AffineConversion=off
  MATLAB Function : MATLAB Function  TreatAsAtomicUnit=on
  Scope : Scope
  Scope1 : Scope
  Simulink-PS Converter7 : nesl_utility/Simulink-PS Converter  PhysicalDomain=network_engine_domain  SubClassName=ps_input  LeftPortType=input  RightPortType=output  PseudoPeriodic=off  Frequencies=[]  NoiseDistribution=none  NoiseParameters=[]  Unit=N*m  AffineConversion=off  InputFiltering=off  SimscapeFilterOrder=1  InputFilterTimeConstant=0.001  UdotUserProvided=1
  Conn1 : PMIOPort  Port=1  Side=Right
  Conn2 : PMIOPort  Port=2  Side=Left
  position : Outport
  wires:
  Conv17/1 -> Scope1/1, MATLAB Function/1(joint), position/1
  MATLAB Function/1(torque) -> Scope/1, Simulink-PS Converter7/1
  connections:
  Ankle Joint2/RConn1 -- Conn2/RConn1
  Ankle Joint2/LConn1 -- Conn1/RConn1
  Conv17/LConn1 -- Ankle Joint2/RConn2
  Simulink-PS Converter7/RConn1 -- Ankle Joint2/LConn2

== system Control_model_10DOF_fin/10DoF Walker SimMechanics Model/Ankle EI1 ==
  Ankle Joint2 : sm_lib/Joints/Revolute Joint  SenseConstraintForce=off  SenseConstraintForceX=off  SenseConstraintForceY=off  SenseConstraintForceZ=off  SenseConstraintTorque=off  SenseConstraintTorqueX=off  SenseConstraintTorqueY=off  SenseConstraintTorqueZ=off  SenseTotalForce=off  SenseTotalForceX=off  SenseTotalForceY=off  SenseTotalForceZ=off  SenseTotalTorque=off  SenseTotalTorqueX=off  SenseTotalTorqueY=off  SenseTotalTorqueZ=off  CompositeWrenchDir=FollowerOnBase  CompositeWrenchFrame=BaseFrame  EquilibriumPosition=0  EquilibriumPositionUnits=deg  SpringStiffness=ankle_stiffness  SpringStiffnessUnits=N*m/rad  DampingCoefficient=joint_damping  DampingCoefficientUnits=N*m/(rad/s)  TorqueActuationMode=InputTorque  MotionActuationMode=ComputedMotion  SensePosition=on  SenseVelocity=off  SenseAcceleration=off  SenseTorqueForce=off  PositionTargetSpecify=on  PositionTargetPriority=High  PositionTargetValue=0  PositionTargetValueUnits=deg  VelocityTargetSpecify=off  VelocityTargetPriority=High  VelocityTargetValue=0  VelocityTargetValueUnits=deg/s
  Conv17 : nesl_utility/PS-Simulink Converter  PhysicalDomain=network_engine_domain  SubClassName=ps_output  LeftPortType=input  RightPortType=output  PseudoPeriodic=off  Frequencies=[]  Unit=rad  AffineConversion=off
  MATLAB Function : MATLAB Function  TreatAsAtomicUnit=on
  Scope : Scope
  Scope1 : Scope
  Simulink-PS Converter7 : nesl_utility/Simulink-PS Converter  PhysicalDomain=network_engine_domain  SubClassName=ps_input  LeftPortType=input  RightPortType=output  PseudoPeriodic=off  Frequencies=[]  NoiseDistribution=none  NoiseParameters=[]  Unit=N*m  AffineConversion=off  InputFiltering=off  SimscapeFilterOrder=1  InputFilterTimeConstant=0.001  UdotUserProvided=1
  Conn1 : PMIOPort  Port=1  Side=Right
  Conn2 : PMIOPort  Port=2  Side=Left
  position : Outport
  wires:
  Conv17/1 -> Scope1/1, MATLAB Function/1(joint), position/1
  MATLAB Function/1(torque) -> Scope/1, Simulink-PS Converter7/1
  connections:
  Ankle Joint2/RConn1 -- Conn2/RConn1
  Ankle Joint2/LConn1 -- Conn1/RConn1
  Conv17/LConn1 -- Ankle Joint2/RConn2
  Simulink-PS Converter7/RConn1 -- Ankle Joint2/LConn2

== system Control_model_10DOF_fin/10DoF Walker SimMechanics Model/Ankle FE ==
  torque : Inport
  Ankle Joint : sm_lib/Joints/Revolute Joint  SenseConstraintForce=off  SenseConstraintForceX=off  SenseConstraintForceY=off  SenseConstraintForceZ=off  SenseConstraintTorque=off  SenseConstraintTorqueX=off  SenseConstraintTorqueY=off  SenseConstraintTorqueZ=off  SenseTotalForce=off  SenseTotalForceX=off  SenseTotalForceY=off  SenseTotalForceZ=off  SenseTotalTorque=off  SenseTotalTorqueX=off  SenseTotalTorqueY=off  SenseTotalTorqueZ=off  CompositeWrenchDir=FollowerOnBase  CompositeWrenchFrame=BaseFrame  EquilibriumPosition=0  EquilibriumPositionUnits=deg  SpringStiffness=0  SpringStiffnessUnits=N*m/rad  DampingCoefficient=joint_damping  DampingCoefficientUnits=N*m/(rad/s)  TorqueActuationMode=InputTorque  MotionActuationMode=ComputedMotion  SensePosition=on  SenseVelocity=on  SenseAcceleration=off  SenseTorqueForce=off  PositionTargetSpecify=on  PositionTargetPriority=High  PositionTargetValue=jointsinitial(1)  PositionTargetValueUnits=rad  VelocityTargetSpecify=off  VelocityTargetPriority=High  VelocityTargetValue=0  VelocityTargetValueUnits=deg/s
  Conv8 : nesl_utility/PS-Simulink Converter  PhysicalDomain=network_engine_domain  SubClassName=ps_output  LeftPortType=input  RightPortType=output  PseudoPeriodic=off  Frequencies=[]  Unit=rad  AffineConversion=off
  Conv9 : nesl_utility/PS-Simulink Converter  PhysicalDomain=network_engine_domain  SubClassName=ps_output  LeftPortType=input  RightPortType=output  PseudoPeriodic=off  Frequencies=[]  Unit=rad/s  AffineConversion=off
  MATLAB Function : MATLAB Function  TreatAsAtomicUnit=on
  Simulink-PS Converter7 : nesl_utility/Simulink-PS Converter  PhysicalDomain=network_engine_domain  SubClassName=ps_input  LeftPortType=input  RightPortType=output  PseudoPeriodic=off  Frequencies=[]  NoiseDistribution=none  NoiseParameters=[]  Unit=N*m  AffineConversion=off  InputFiltering=off  SimscapeFilterOrder=1  InputFilterTimeConstant=0.001  UdotUserProvided=1
  Conn1 : PMIOPort  Port=1  Side=Left
  Conn2 : PMIOPort  Port=2  Side=Right
  position : Outport
  velocity : Outport  Port=2
  wires:
  Conv8/1 -> MATLAB Function/1(joint), position/1
  Conv9/1 -> MATLAB Function/2(velocity), velocity/1
  MATLAB Function/1(torque) -> Simulink-PS Converter7/1
  torque/1 -> MATLAB Function/3(desired_torque)
  connections:
  Ankle Joint/LConn1 -- Conn2/RConn1
  Conv8/LConn1 -- Ankle Joint/RConn2
  Ankle Joint/LConn2 -- Simulink-PS Converter7/RConn1
  Conv9/LConn1 -- Ankle Joint/RConn3
  Conn1/RConn1 -- Ankle Joint/RConn1
